simulink model "temperature_change"  (R2022a)
settings: Solver=VariableStepAuto  StartTime=0.0  StopTime=10.0  RelTol=1e-3
settings Model: Creator=Amogh  LastModifiedBy=Amogh

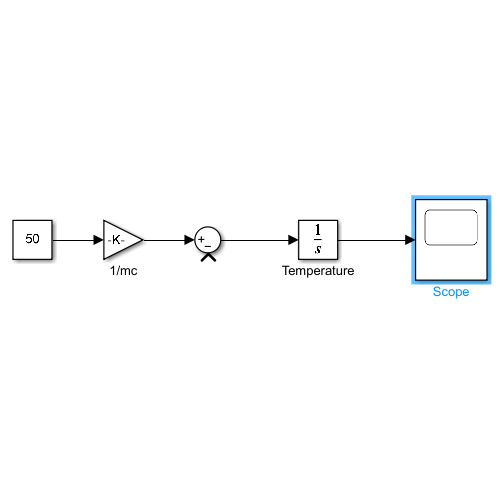
[thumbnail: Simulink's stored preview of the top-level diagram]
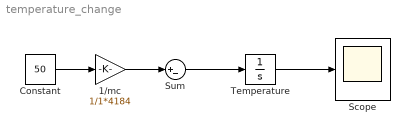
== system temperature_change ==
  1/mc : Gain  Gain=1/1*4184
  Constant : Constant  Value=50
  Scope : Scope
  Sum : Sum  Inputs=|+-
  Temperature : Integrator
  wires:
  Constant/1 -> 1/mc/1
  Temperature/1 -> Scope/1
  1/mc/1 -> Sum/1
  Sum/1 -> Temperature/1
